simulink model "Quadcopter_Dynamics_Model"  (R2023a)
settings: Solver=ode4  StartTime=0.0  StopTime=5  FixedStep=0.001  RelTol=1e-3
settings Model: Creator=玖辞丶  LastModifiedBy=16282
settings SolverCC: AlgebraicLoopSolver=TrustRegion
settings DataIOCC: ReturnWorkspaceOutputs=off
settings OptimizationCC: ReuseModelBlockBuffer=off
settings DebuggingCC: UnconnectedInputMsg=warning  UnconnectedOutputMsg=warning  UnconnectedLineMsg=warning  ArithmeticOperatorsInVariantConditions=warning
settings ModelReferenceCC: EnableRefExpFcnMdlSchedulingChecks=on
settings SFSimCC: CustomCodeUndefinedFunction=UseInterfaceOnly

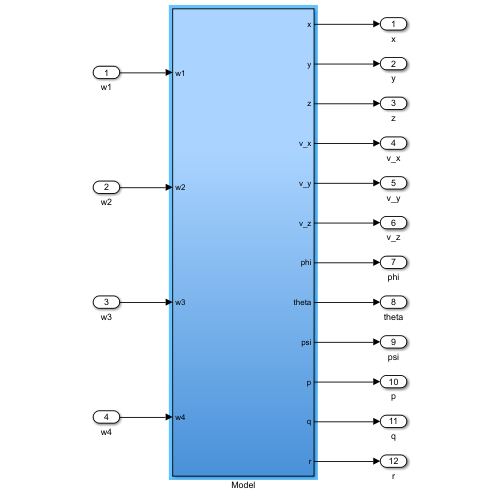
[thumbnail: Simulink's stored preview of the top-level diagram]
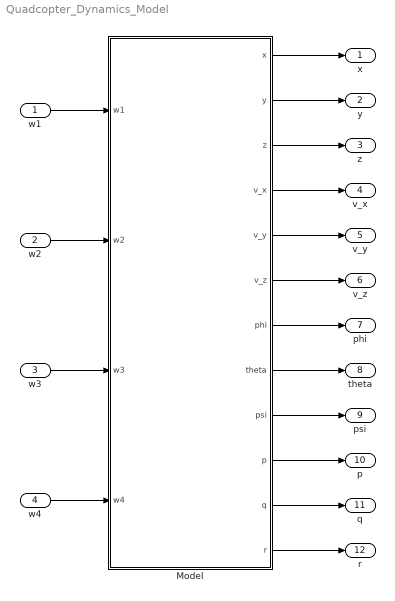
== system Quadcopter_Dynamics_Model ==
  w1 : Inport
  w2 : Inport  Port=2
  w3 : Inport  Port=3
  w4 : Inport  Port=4
  Model : Subsystem
  x : Outport
  y : Outport  Port=2
  z : Outport  Port=3
  v_x : Outport  Port=4
  v_y : Outport  Port=5
  v_z : Outport  Port=6
  phi : Outport  Port=7
  theta : Outport  Port=8
  psi : Outport  Port=9
  p : Outport  Port=10
  q : Outport  Port=11
  r : Outport  Port=12
  wires:
  w1/1 -> Model/1(w1)
  w2/1 -> Model/2(w2)
  w3/1 -> Model/3(w3)
  w4/1 -> Model/4(w4)
  Model/1(x) -> x/1
  Model/2(y) -> y/1
  Model/3(z) -> z/1
  Model/4(v_x) -> v_x/1
  Model/5(v_y) -> v_y/1
  Model/6(v_z) -> v_z/1
  Model/7(phi) -> phi/1
  Model/8(theta) -> theta/1
  Model/9(psi) -> psi/1
  Model/10(p) -> p/1
  Model/11(q) -> q/1
  Model/12(r) -> r/1

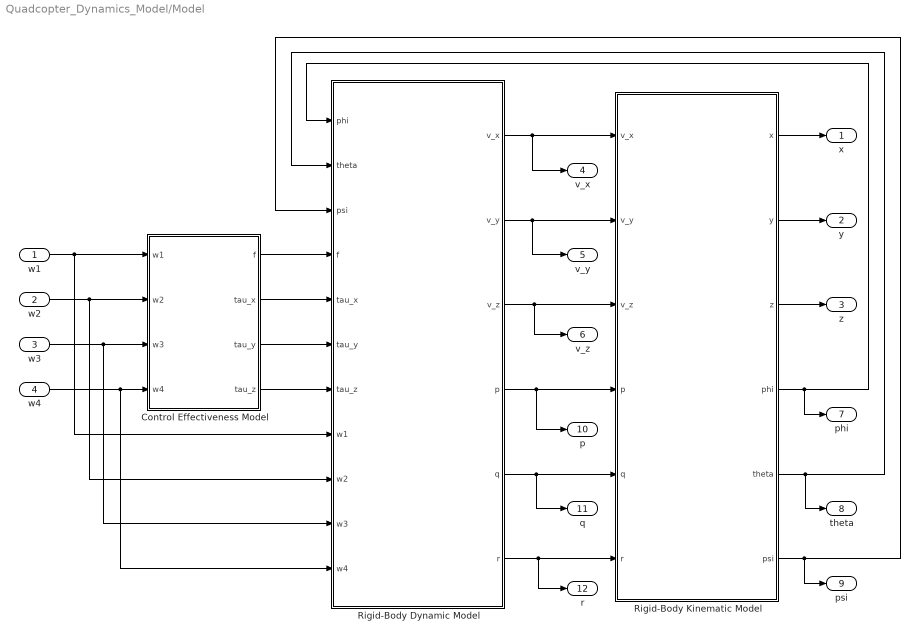
== system Quadcopter_Dynamics_Model/Model ==
  w1 : Inport
  w2 : Inport  Port=2
  w3 : Inport  Port=3
  w4 : Inport  Port=4
  Control Effectiveness Model : Subsystem
  Rigid-Body Dynamic Model : Subsystem
  Rigid-Body Kinematic Model : Subsystem
  x : Outport  VectorParamsAs1DForOutWhenUnconnected=off
  y : Outport  Port=2  VectorParamsAs1DForOutWhenUnconnected=off
  z : Outport  Port=3  VectorParamsAs1DForOutWhenUnconnected=off
  v_x : Outport  Port=4  VectorParamsAs1DForOutWhenUnconnected=off
  v_y : Outport  Port=5  VectorParamsAs1DForOutWhenUnconnected=off
  v_z : Outport  Port=6  VectorParamsAs1DForOutWhenUnconnected=off
  phi : Outport  Port=7  VectorParamsAs1DForOutWhenUnconnected=off
  theta : Outport  Port=8  VectorParamsAs1DForOutWhenUnconnected=off
  psi : Outport  Port=9  VectorParamsAs1DForOutWhenUnconnected=off
  p : Outport  Port=10  VectorParamsAs1DForOutWhenUnconnected=off
  q : Outport  Port=11  VectorParamsAs1DForOutWhenUnconnected=off
  r : Outport  Port=12  VectorParamsAs1DForOutWhenUnconnected=off
  wires:
  w1/1 -> Rigid-Body Dynamic Model/8(w1), Control Effectiveness Model/1(w1)
  Control Effectiveness Model/1(f) -> Rigid-Body Dynamic Model/4(f)
  w3/1 -> Rigid-Body Dynamic Model/10(w3), Control Effectiveness Model/3(w3)
  Rigid-Body Kinematic Model/5(theta) -> theta/1, Rigid-Body Dynamic Model/2(theta)
  w4/1 -> Rigid-Body Dynamic Model/11(w4), Control Effectiveness Model/4(w4)
  Rigid-Body Kinematic Model/4(phi) -> Rigid-Body Dynamic Model/1(phi), phi/1
  w2/1 -> Rigid-Body Dynamic Model/9(w2), Control Effectiveness Model/2(w2)
  Rigid-Body Dynamic Model/4(p) -> Rigid-Body Kinematic Model/4(p), p/1
  Rigid-Body Dynamic Model/3(v_z) -> Rigid-Body Kinematic Model/3(v_z), v_z/1
  Rigid-Body Dynamic Model/6(r) -> Rigid-Body Kinematic Model/6(r), r/1
  Control Effectiveness Model/2(tau_x) -> Rigid-Body Dynamic Model/5(tau_x)
  Rigid-Body Dynamic Model/2(v_y) -> Rigid-Body Kinematic Model/2(v_y), v_y/1
  Rigid-Body Kinematic Model/1(x) -> x/1
  Rigid-Body Kinematic Model/6(psi) -> psi/1, Rigid-Body Dynamic Model/3(psi)
  Rigid-Body Dynamic Model/5(q) -> Rigid-Body Kinematic Model/5(q), q/1
  Control Effectiveness Model/4(tau_z) -> Rigid-Body Dynamic Model/7(tau_z)
  Rigid-Body Kinematic Model/2(y) -> y/1
  Rigid-Body Kinematic Model/3(z) -> z/1
  Rigid-Body Dynamic Model/1(v_x) -> v_x/1, Rigid-Body Kinematic Model/1(v_x)
  Control Effectiveness Model/3(tau_y) -> Rigid-Body Dynamic Model/6(tau_y)

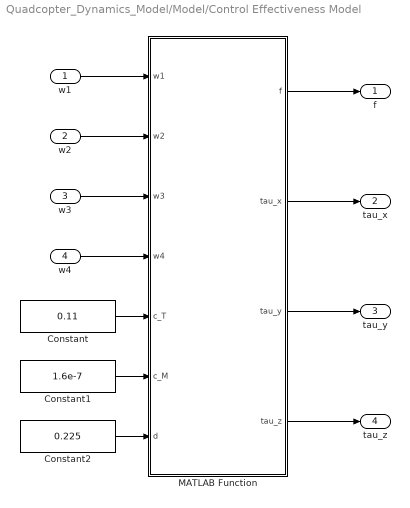
== system Quadcopter_Dynamics_Model/Model/Control Effectiveness Model ==
  w1 : Inport
  w2 : Inport  Port=2
  w3 : Inport  Port=3
  w4 : Inport  Port=4
  Constant : Constant  Value=0.11
  Constant1 : Constant  Value=1.6e-7
  Constant2 : Constant  Value=0.225
  MATLAB Function : MATLAB Function  TreatAsAtomicUnit=on
  f : Outport  VectorParamsAs1DForOutWhenUnconnected=off
  tau_x : Outport  Port=2  VectorParamsAs1DForOutWhenUnconnected=off
  tau_y : Outport  Port=3  VectorParamsAs1DForOutWhenUnconnected=off
  tau_z : Outport  Port=4  VectorParamsAs1DForOutWhenUnconnected=off
  wires:
  Constant1/1 -> MATLAB Function/6(c_M)
  Constant/1 -> MATLAB Function/5(c_T)
  MATLAB Function/3(tau_y) -> tau_y/1
  MATLAB Function/1(f) -> f/1
  Constant2/1 -> MATLAB Function/7(d)
  MATLAB Function/4(tau_z) -> tau_z/1
  w3/1 -> MATLAB Function/3(w3)
  w1/1 -> MATLAB Function/1(w1)
  w4/1 -> MATLAB Function/4(w4)
  MATLAB Function/2(tau_x) -> tau_x/1
  w2/1 -> MATLAB Function/2(w2)

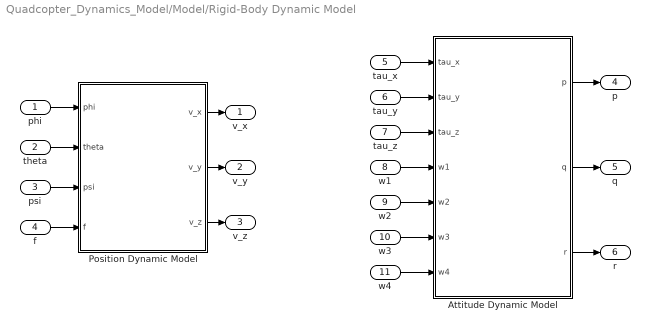
== system Quadcopter_Dynamics_Model/Model/Rigid-Body Dynamic Model ==
  phi : Inport
  theta : Inport  Port=2
  psi : Inport  Port=3
  f : Inport  Port=4
  tau_x : Inport  Port=5
  tau_y : Inport  Port=6
  tau_z : Inport  Port=7
  w1 : Inport  Port=8
  w2 : Inport  Port=9
  w3 : Inport  Port=10
  w4 : Inport  Port=11
  Attitude Dynamic Model : Subsystem
  Position Dynamic Model : Subsystem
  v_x : Outport  VectorParamsAs1DForOutWhenUnconnected=off
  v_y : Outport  Port=2  VectorParamsAs1DForOutWhenUnconnected=off
  v_z : Outport  Port=3  VectorParamsAs1DForOutWhenUnconnected=off
  p : Outport  Port=4  VectorParamsAs1DForOutWhenUnconnected=off
  q : Outport  Port=5  VectorParamsAs1DForOutWhenUnconnected=off
  r : Outport  Port=6  VectorParamsAs1DForOutWhenUnconnected=off
  wires:
  w3/1 -> Attitude Dynamic Model/6(w3)
  w1/1 -> Attitude Dynamic Model/4(w1)
  theta/1 -> Position Dynamic Model/2(theta)
  f/1 -> Position Dynamic Model/4(f)
  tau_x/1 -> Attitude Dynamic Model/1(tau_x)
  w2/1 -> Attitude Dynamic Model/5(w2)
  Attitude Dynamic Model/1(p) -> p/1
  w4/1 -> Attitude Dynamic Model/7(w4)
  Attitude Dynamic Model/2(q) -> q/1
  tau_y/1 -> Attitude Dynamic Model/2(tau_y)
  tau_z/1 -> Attitude Dynamic Model/3(tau_z)
  Position Dynamic Model/3(v_z) -> v_z/1
  Attitude Dynamic Model/3(r) -> r/1
  phi/1 -> Position Dynamic Model/1(phi)
  psi/1 -> Position Dynamic Model/3(psi)
  Position Dynamic Model/1(v_x) -> v_x/1
  Position Dynamic Model/2(v_y) -> v_y/1

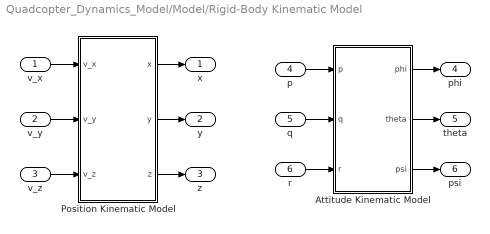
== system Quadcopter_Dynamics_Model/Model/Rigid-Body Kinematic Model ==
  v_x : Inport
  v_y : Inport  Port=2
  v_z : Inport  Port=3
  p : Inport  Port=4
  q : Inport  Port=5
  r : Inport  Port=6
  Attitude Kinematic Model : Subsystem
  Position Kinematic Model : Subsystem
  x : Outport  VectorParamsAs1DForOutWhenUnconnected=off
  y : Outport  Port=2  VectorParamsAs1DForOutWhenUnconnected=off
  z : Outport  Port=3  VectorParamsAs1DForOutWhenUnconnected=off
  phi : Outport  Port=4  VectorParamsAs1DForOutWhenUnconnected=off
  theta : Outport  Port=5  VectorParamsAs1DForOutWhenUnconnected=off
  psi : Outport  Port=6  VectorParamsAs1DForOutWhenUnconnected=off
  wires:
  v_x/1 -> Position Kinematic Model/1(v_x)
  v_y/1 -> Position Kinematic Model/2(v_y)
  r/1 -> Attitude Kinematic Model/3(r)
  p/1 -> Attitude Kinematic Model/1(p)
  v_z/1 -> Position Kinematic Model/3(v_z)
  Position Kinematic Model/1(x) -> x/1
  Position Kinematic Model/2(y) -> y/1
  q/1 -> Attitude Kinematic Model/2(q)
  Position Kinematic Model/3(z) -> z/1
  Attitude Kinematic Model/2(theta) -> theta/1
  Attitude Kinematic Model/1(phi) -> phi/1
  Attitude Kinematic Model/3(psi) -> psi/1

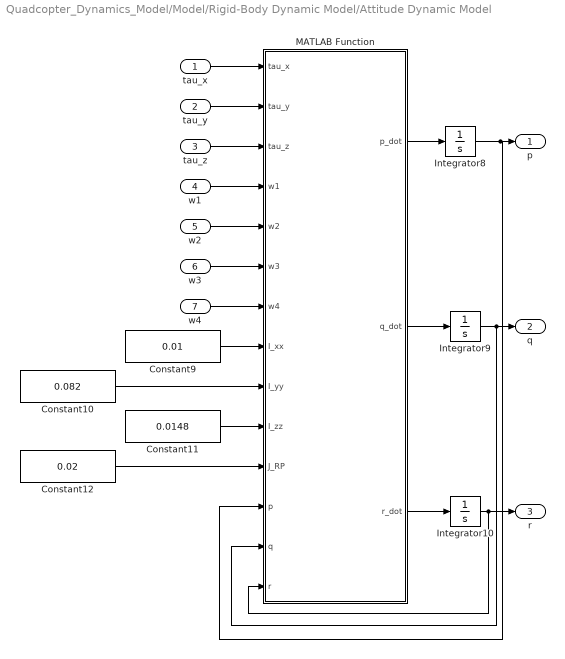
== system Quadcopter_Dynamics_Model/Model/Rigid-Body Dynamic Model/Attitude Dynamic Model ==
  tau_x : Inport
  tau_y : Inport  Port=2
  tau_z : Inport  Port=3
  w1 : Inport  Port=4
  w2 : Inport  Port=5
  w3 : Inport  Port=6
  w4 : Inport  Port=7
  Constant10 : Constant  Value=0.082
  Constant11 : Constant  Value=0.0148
  Constant12 : Constant  Value=0.02
  Constant9 : Constant  Value=0.01
  Integrator10 : Integrator
  Integrator8 : Integrator
  Integrator9 : Integrator
  MATLAB Function : MATLAB Function  TreatAsAtomicUnit=on
  p : Outport  VectorParamsAs1DForOutWhenUnconnected=off
  q : Outport  Port=2  VectorParamsAs1DForOutWhenUnconnected=off
  r : Outport  Port=3  VectorParamsAs1DForOutWhenUnconnected=off
  wires:
  Integrator10/1 -> r/1, MATLAB Function/14(r)
  Integrator9/1 -> MATLAB Function/13(q), q/1
  MATLAB Function/3(r_dot) -> Integrator10/1
  MATLAB Function/1(p_dot) -> Integrator8/1
  Integrator8/1 -> MATLAB Function/12(p), p/1
  MATLAB Function/2(q_dot) -> Integrator9/1
  tau_x/1 -> MATLAB Function/1(tau_x)
  tau_y/1 -> MATLAB Function/2(tau_y)
  tau_z/1 -> MATLAB Function/3(tau_z)
  w1/1 -> MATLAB Function/4(w1)
  w2/1 -> MATLAB Function/5(w2)
  w3/1 -> MATLAB Function/6(w3)
  w4/1 -> MATLAB Function/7(w4)
  Constant9/1 -> MATLAB Function/8(I_xx)
  Constant10/1 -> MATLAB Function/9(I_yy)
  Constant11/1 -> MATLAB Function/10(I_zz)
  Constant12/1 -> MATLAB Function/11(J_RP)

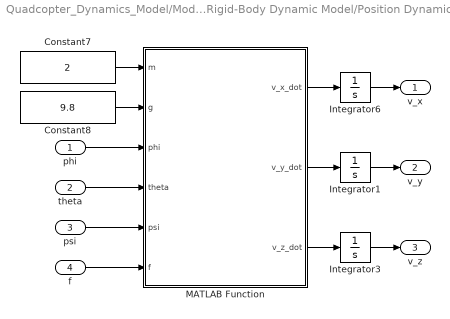
== system Quadcopter_Dynamics_Model/Model/Rigid-Body Dynamic Model/Position Dynamic Model ==
  phi : Inport
  theta : Inport  Port=2
  psi : Inport  Port=3
  f : Inport  Port=4
  Constant7 : Constant  Value=2
  Constant8 : Constant  Value=9.8
  Integrator1 : Integrator
  Integrator3 : Integrator
  Integrator6 : Integrator
  MATLAB Function : MATLAB Function  TreatAsAtomicUnit=on
  v_x : Outport  VectorParamsAs1DForOutWhenUnconnected=off
  v_y : Outport  Port=2  VectorParamsAs1DForOutWhenUnconnected=off
  v_z : Outport  Port=3  VectorParamsAs1DForOutWhenUnconnected=off
  wires:
  Constant8/1 -> MATLAB Function/2(g)
  MATLAB Function/1(v_x_dot) -> Integrator6/1
  MATLAB Function/2(v_y_dot) -> Integrator1/1
  theta/1 -> MATLAB Function/4(theta)
  Constant7/1 -> MATLAB Function/1(m)
  MATLAB Function/3(v_z_dot) -> Integrator3/1
  phi/1 -> MATLAB Function/3(phi)
  f/1 -> MATLAB Function/6(f)
  psi/1 -> MATLAB Function/5(psi)
  Integrator6/1 -> v_x/1
  Integrator1/1 -> v_y/1
  Integrator3/1 -> v_z/1

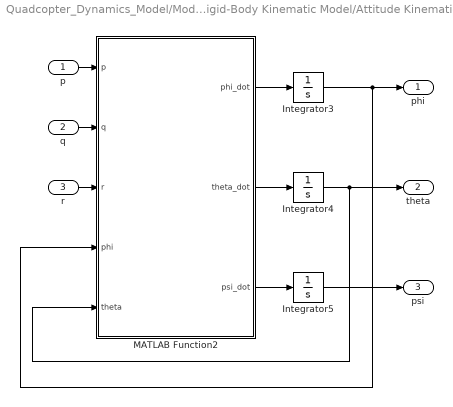
== system Quadcopter_Dynamics_Model/Model/Rigid-Body Kinematic Model/Attitude Kinematic Model ==
  p : Inport
  q : Inport  Port=2
  r : Inport  Port=3
  Integrator3 : Integrator
  Integrator4 : Integrator
  Integrator5 : Integrator
  MATLAB Function2 : MATLAB Function  TreatAsAtomicUnit=on
  phi : Outport  VectorParamsAs1DForOutWhenUnconnected=off
  theta : Outport  Port=2  VectorParamsAs1DForOutWhenUnconnected=off
  psi : Outport  Port=3  VectorParamsAs1DForOutWhenUnconnected=off
  wires:
  r/1 -> MATLAB Function2/3(r)
  MATLAB Function2/1(phi_dot) -> Integrator3/1
  q/1 -> MATLAB Function2/2(q)
  Integrator3/1 -> phi/1, MATLAB Function2/4(phi)
  Integrator4/1 -> theta/1, MATLAB Function2/5(theta)
  Integrator5/1 -> psi/1
  p/1 -> MATLAB Function2/1(p)
  MATLAB Function2/3(psi_dot) -> Integrator5/1
  MATLAB Function2/2(theta_dot) -> Integrator4/1

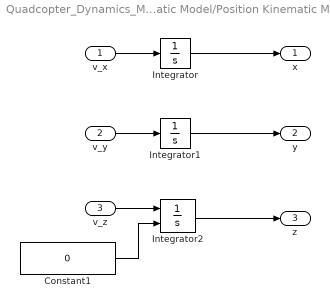
== system Quadcopter_Dynamics_Model/Model/Rigid-Body Kinematic Model/Position Kinematic Model ==
  v_x : Inport
  v_y : Inport  Port=2
  v_z : Inport  Port=3
  Constant1 : Constant  Value=0
  Integrator : Integrator
  Integrator1 : Integrator
  Integrator2 : Integrator  InitialConditionSource=external
  x : Outport  VectorParamsAs1DForOutWhenUnconnected=off
  y : Outport  Port=2  VectorParamsAs1DForOutWhenUnconnected=off
  z : Outport  Port=3  VectorParamsAs1DForOutWhenUnconnected=off
  wires:
  v_z/1 -> Integrator2/1
  Integrator1/1 -> y/1
  Integrator/1 -> x/1
  Constant1/1 -> Integrator2/2
  Integrator2/1 -> z/1
  v_x/1 -> Integrator/1
  v_y/1 -> Integrator1/1

== matlab function Quadcopter_Dynamics_Model/Model/Rigid-Body Kinematic Model/Attitude Kinematic Model/MATLAB Function2 ==
  data: p input; phi_dot output; q input; r input; phi input; theta input; theta_dot output; psi_dot output
% 函数描述
% 1.作用：本函数为四旋翼的姿态运动学微分方程组，通过四旋翼的机体角速度计算得到四旋翼的姿态角

function [phi_dot, theta_dot, psi_dot] = fcn(p, q, r, phi, theta)
    
    % 2.函数输入：
    %   p：四旋翼x轴角速度（机体轴)(rad/s)
    %   q：四旋翼y轴角速度（机体轴)(rad/s)
    %   r：四旋翼z轴角速度（机体轴)(rad/s)
    %   phi：滚转角(rad)
    %   theta：俯仰角(rad)

    %   phi_dot：滚转角速度
    phi_dot = p + q * tan(theta) * sin(phi) + r * tan(theta) * cos(phi);

    %   theta_dot：俯仰角速度
    theta_dot = q * cos(phi) - r * sin(phi);

    %   psi_dot：偏航角速度
    psi_dot = (q * sin(phi) + r * cos(phi)) / cos(theta);

end

== matlab function Quadcopter_Dynamics_Model/Model/Control Effectiveness Model/MATLAB Function ==
  data: w1 input; f output; w2 input; w3 input; w4 input; c_T input; c_M input; d input; tau_x output; tau_y output; tau_z output
% 函数描述
% 1.作用：本函数用来计算螺旋桨旋转产生的总拉力和反扭力矩。

function [f, tau_x, tau_y, tau_z] = fcn(w1, w2, w3, w4, c_T, c_M, d)

% 2.函数输入：
%   wi：四个螺旋桨的转速(rad/s)
%   c_T：螺旋桨拉力系数
%   c_M：螺旋桨转矩系数
%   d：机体中心和任一电机的距离(m)

% 3.函数输出：
%   f：螺旋桨拉力（机体轴）
%   tau_x：x轴反扭力矩（机体轴）
%   tau_y：y轴反扭力矩（机体轴）
%   tau_z：z轴反扭力矩（机体轴）

    f = c_T * (w1^2 + w2^2 + w3^2 + w4^2);
    tau_x = d * c_T * (sqrt(2)/2) * (-w1^2 + w2^2 + w3^2 - w4^2);
    tau_y = d * c_T * (sqrt(2)/2) * (w1^2 - w2^2 + w3^2 - w4^2);
    tau_z = c_M * (w1^2 + w2^2 - w3^2 - w4^2);
    
end

== matlab function Quadcopter_Dynamics_Model/Model/Rigid-Body Dynamic Model/Position Dynamic Model/MATLAB Function ==
  data: m input; g input; phi input; theta input; psi input; f input; v_x_dot output; v_y_dot output; v_z_dot output
% 函数描述
% 1.作用：本函数为四旋翼的位置动力学微分方程组，通过四旋翼所受拉力、姿态角计算得到四旋翼飞行器的加速度

function [v_x_dot, v_y_dot, v_z_dot] = fcn(m, g, phi, theta, psi, f)

    % 2.函数输入：
    %   m：四旋翼飞行器质量(kg)
    %   g：重力加速度(m/s^2)
    %   phi：滚转角(rad)
    %   theta：俯仰角(rad)
    %   psi：偏航角(rad)
    %   f：螺旋桨产生的总拉力(N)
    
    %   v_x_dot：地球坐标系下沿x轴的速度的导数
    v_x_dot = -f * (1/m) * (cos(psi) * sin(theta) * cos(phi) + sin(psi) * sin(phi));
    
    %   v_y_dot：地球坐标系下沿y轴的速度的导数
    v_y_dot = -f * (1/m) * (sin(psi) * sin(theta) * cos(phi) - cos(psi) * sin(phi));
    
    %   v_z_dot：地球坐标系下沿z轴的速度的导数
    v_z_dot = g - f * (1/m) * cos(phi) * cos(theta);

end

== matlab function Quadcopter_Dynamics_Model/Model/Rigid-Body Dynamic Model/Attitude Dynamic Model/MATLAB Function ==
  data: p_dot output; q_dot output; r_dot output; tau_x input; tau_y input; tau_z input; w1 input; w2 input; w3 input; w4 input; I_xx input; I_yy input; I_zz input; J_RP input; p input; q input; r input
% 函数描述
% 1.作用：本函数为四旋翼的姿态动力学微分方程组，通过四旋翼所受力矩和螺旋桨转速计算得到四旋翼的机体角速度

function [p_dot, q_dot, r_dot] = ...
fcn(tau_x, tau_y, tau_z, w1, w2, w3, w4, I_xx, I_yy, I_zz, J_RP, p, q, r)
    
    % 2.函数输入：
    %   wi：四个螺旋桨的转速(rad/s)
    %   tau_x：x轴反扭力矩（机体轴）(N·m)
    %   tau_y：y轴反扭力矩（机体轴）(N·m)
    %   tau_z：z轴反扭力矩（机体轴）(N·m)
    %   I_xx：四旋翼x轴转动惯量(kg·m^2)
    %   I_yy：四旋翼y轴转动惯量(kg·m^2)
    %   I_zz：四旋翼z轴转动惯量(kg·m^2)
    %   J_RP：整个电机转子和螺旋桨绕转轴的总转动惯量(kg·m^2)
  
    Omega = -w1 + w2 - w3 + w4;

    %   p_dot：四旋翼x轴角加速度（机体轴)
    %   p：四旋翼x轴角速度（机体轴)(rad/s)
    p_dot = (1/I_xx) * (tau_x + q * r * (I_yy - I_zz) - J_RP * q * Omega);

    %   q_dot：四旋翼y轴角加速度（机体轴)
    %   q：四旋翼y轴角速度（机体轴)(rad/s)
    q_dot = (1/I_yy) * (tau_y + p * r * (I_zz - I_xx) + J_RP * p * Omega);

    %   r_dot：四旋翼z轴角加速度（机体轴)
    %   r：四旋翼z轴角速度（机体轴)(rad/s)
    r_dot = (1/I_zz) * (tau_z + p * q * (I_xx - I_yy) );

end
